simulink model "coord_rotations_test"  (R2016b)
settings: Solver=VariableStepAuto  StartTime=0.0  StopTime=1  RelTol=1e-3
values from neighbouring files (symbols this model uses):
  JD = 2453101.827396 + sec_2_JD*s_frac    (= 2453101.82741)    [coord_rot_time_test_init.m]
  JD_2_cent = 1/(36525)    (= 2.73785078713e-05)    [coord_rot_time_test_init.m]
  JD_tt_cent = 0.0426236319    [coord_rot_time_test_init.m]
  JD_ut1_cent = JD_2_cent*(JD - JD_J2000)    (= 0.0426236114155)    [coord_rot_time_test_init.m]
  rECI = [ -1033.4793830; 7901.2952754; 6380.3565958 ]    [coord_rot_time_test_init.m]
  rTEME = [ -9060.47373569; 4658.70952502; 813.68673153 ]    [coord_rot_time_test_init.m]
  sec_2_cent = 1/(86400*36525)    (= 3.1688087814e-10)    [coord_rot_time_test_init.m]
  ut1_2_tt = 32.184 + 32 + dut1    (= 64.388241)    [coord_rot_time_test_init.m]
  vECI = [ -3.225636520; -2.872451450; 5.531924446 ]    [coord_rot_time_test_init.m]
  vTEME = [ -2.232832783; -4.110453490; -3.157345433 ]    [coord_rot_time_test_init.m]
libraries: coord_rotation_lib x2
settings Model: Creator=taylorreynolds  LastModifiedBy=taylorreynolds

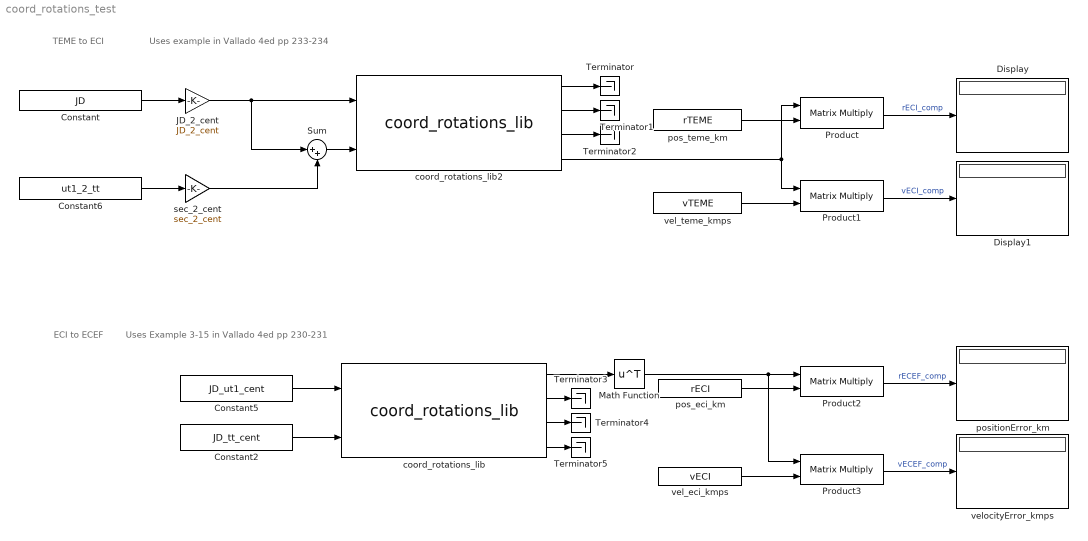
== system coord_rotations_test ==
  note: Uses Example 3-15 in Vallado 4ed pp 230-231
  note: Uses example in Vallado 4ed pp 233-234
  note: ECI to ECEF
  note: TEME to ECI
  Constant : Constant  Value=JD
  Constant2 : Constant  Value=JD_tt_cent
  Constant5 : Constant  Value=JD_ut1_cent
  Constant6 : Constant  Value=ut1_2_tt
  Display : Display
  Display1 : Display
  JD_2_cent : Gain  Gain=JD_2_cent
  Math Function : Math  Operator=transpose  SaturateOnIntegerOverflow=on
  Product{,1..3} (4 alike) : Product  Multiplication=Matrix(*)
  Sum : Sum  Inputs=|++
  Terminator{,1..5} (6 alike) : Terminator
  coord_rotations_lib : coord_rotation_lib/coord_rotations_lib
  coord_rotations_lib2 : coord_rotation_lib/coord_rotations_lib
  pos_eci_km : Constant  Value=rECI
  pos_teme_km : Constant  Value=rTEME
  positionError_km : Display
  sec_2_cent : Gain  Gain=sec_2_cent
  vel_eci_kmps : Constant  Value=vECI
  vel_teme_kmps : Constant  Value=vTEME
  velocityError_kmps : Display
  wires:
  Constant/1 -> JD_2_cent/1
  JD_2_cent/1 -> coord_rotations_lib2/1, Sum/1
  sec_2_cent/1 -> Sum/2
  Sum/1 -> coord_rotations_lib2/2
  coord_rotations_lib2/1 -> Terminator/1
  coord_rotations_lib2/3 -> Terminator2/1
  coord_rotations_lib2/2 -> Terminator1/1
  coord_rotations_lib2/4 -> Product/1, Product1/1
  pos_teme_km/1 -> Product/2
  vel_teme_kmps/1 -> Product1/2
  Product/1 -> Display/1  "rECI_comp"
  Product1/1 -> Display1/1  "vECI_comp"
  Constant2/1 -> coord_rotations_lib/2
  Constant5/1 -> coord_rotations_lib/1
  pos_eci_km/1 -> Product2/2
  vel_eci_kmps/1 -> Product3/2
  Product2/1 -> positionError_km/1  "rECEF_comp"
  coord_rotations_lib/2 -> Terminator3/1
  coord_rotations_lib/3 -> Terminator4/1
  coord_rotations_lib/4 -> Terminator5/1
  Product3/1 -> velocityError_kmps/1  "vECEF_comp"
  Constant6/1 -> sec_2_cent/1
  coord_rotations_lib/1 -> Math Function/1
  Math Function/1 -> Product3/1, Product2/1
